simulink model "OtterFullForLqr_PositionControl_KALMAN"  (R2020b)
settings: Solver=ode4  StartTime=0.0  StopTime=100  FixedStep=0.01  RelTol=1e-3
model workspace (MAT data in the model file):
  count = 1
values from neighbouring files (symbols this model uses):
  u0 = [60 60]'    [LinMod60rpmForLqr.m]
  x0 = OpTrim60.states.x    [LinMod60rpmForLqr.m]
undefined symbols (not defined in the file or in its folder): F, N
libraries: mssSimulink x2, simulink x1
settings Model: Creator=rapha  LastModifiedBy=rapha
settings DataIOCC: ExternalInput=getinputstruct(op_trim1)  InitialState=getstatestruct(op_trim1)

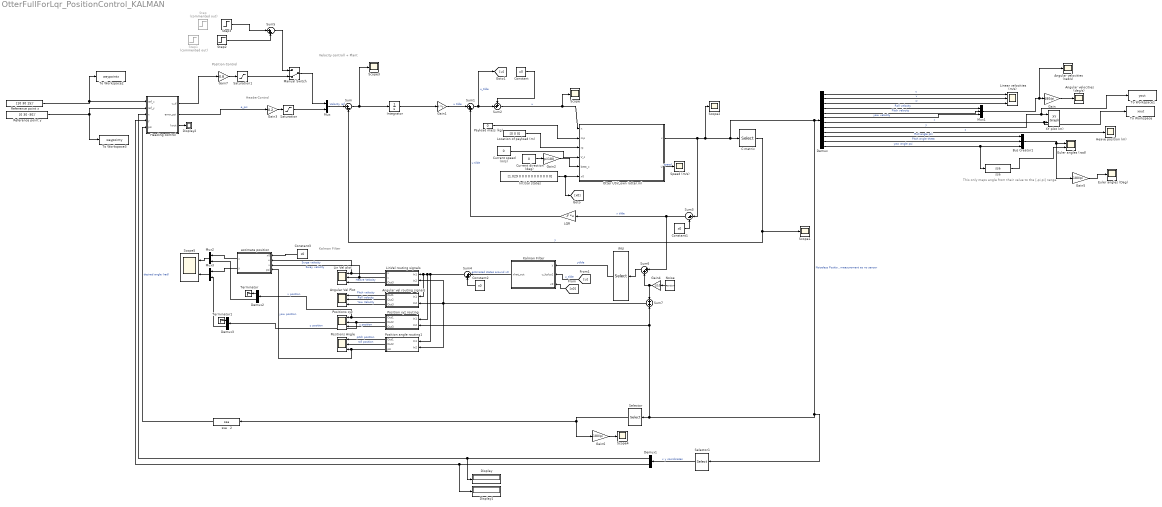
== system OtterFullForLqr_PositionControl_KALMAN ==
  note: Kalman Filter
  note: Position Control
  note: Velocity controll + Plant
  note: This only maps angle from their value to the [-pi,pi] range.
  note: HeaderControl
  Angular Vel Plot : Scope  NumInputPorts=3
  Angular vel routing signals : Subsystem
  Angular velocities (deg/s) : Scope
  Angular velocities (rad/s) : Scope
  Bus Creator1 : BusCreator  Inputs=3
  C matrix : Selector  InputPortWidth=12  IndexOptions=Index vector (dialog)  Indices=[1 6]  OutputSizes=1
  Constant : Constant  Value=u0
  Constant1 : Constant  Value=x0
  Constant2 : Constant  Value=x0
  Constant3 : Constant  Value=x0
  Current direction (deg) : Constant  Value=0
  Current speed (m/s) : Constant  Value=0
  Demux : Demux  Outputs=12
  Demux1 : Demux  Outputs=2
  Demux2 : Demux  Outputs=2
  Demux3 : Demux  Outputs=2
  Display : Display
  Display1 : Display
  Display2 : Display
  Euler angles (Deg) : Scope
  Euler angles (rad) : Scope  NumInputPorts=2
  Gain : Gain  Gain=180/pi
  Gain1 : Gain  Gain=N  Multiplication=Matrix(K*u)
  Gain2 : Gain  Gain=pi/180
  Gain3 : Gain  Gain=0.2
  Gain4 : Gain  Gain=1/10
  Gain5 : Gain  Gain=180/pi
  Gain6 : Gain  Gain=180/pi
  Gain7 : Gain  Gain=0.8
  Heading control : MATLAB Function  TreatAsAtomicUnit=on
  Heave position (m) : Scope
  IMU : Selector  InputPortWidth=12  IndexOptions=Index vector (dialog)  Indices=[1 2 3 4 5 6 10 11 12]  OutputSizes=1
  Integrator : Integrator
  Intitial states : Constant  Value=[1.029 0 0 0 0 0 0 0 0 0 0 0]
  Kalman Filter : MATLAB Function  TreatAsAtomicUnit=on
  LQR : Gain  Gain=-F  Multiplication=Matrix(K*u)
  Lin Vel plot : Scope  NumInputPorts=3
  LinVel routing signals : Subsystem
  Linear velocities (m/s) : Scope  NumInputPorts=3
  Location of payload (m) : Constant  Value=[0 0 0]
  Manual Switch : ManualSwitch  CurrentSetting=0
  Mux : Mux  Inputs=2
  Mux1 : Mux  Inputs=3
  Mux2 : Mux  Inputs=2
  Mux3 : Mux  Inputs=2
  Noise : RandomNumber  Variance=0.01  SampleTime=0.01
  "Otter USV_own (otter.m) " : Subsystem  AncestorBlock=mssSimulink/Marine craft models/Otter USV (otter.m)
      mask Display: image('otter.jpg'); % Use "Edit Image" on toolstrip to change.
  Payload mass (kg) : Constant  Value=0
  Position angle routing1 : Subsystem
  Position xyz routing : Subsystem
  Positions Angle : Scope  NumInputPorts=3
  Positions xyz : Scope  NumInputPorts=3
  Reference point x : Constant  Value=[10 30 15]'
  Reference point y : Constant  Value=[0 30 -30]'
  Saturation : Saturate
  Saturation1 : Saturate  UpperLimit=1.5  LowerLimit=-1.5
  Scope{,1..4} (5 alike) : Scope
  Scope5 : Scope  NumInputPorts=2
  Selector : Selector  InputPortWidth=12  IndexOptions=Index vector (dialog)  Indices=[12]  OutputSizes=1
  Selector1 : Selector  InputPortWidth=12  IndexOptions=Index vector (dialog)  Indices=[7 8]  OutputSizes=1
  Speed (m/s) : Scope
  Step : Step  Commented=on  Before=0.5  After=0.5  SampleTime=0
  Step1 : Step  Commented=on  After=90  SampleTime=0
  Step2 : Step  Time=10  Before=1.029  After=0.8  SampleTime=0
  Step3 : Step  Time=15  After=0.3  SampleTime=0
  Sum : Sum  Inputs=|+-
  Sum{1,4..6} (4 alike) : Sum  Inputs=|++
  Sum2 : Sum  Inputs=++|
  Sum3 : Sum  Inputs=|+-
  Sum7 : Sum  Inputs=+|+
  Terminator : Terminator
  Terminator1 : Terminator
  To Workspace : ToWorkspace  VariableName=xout  SampleTime=-1
  To Workspace1 : ToWorkspace  VariableName=yout  SampleTime=-1
  To Workspace2 : ToWorkspace  VariableName=waypointx  SampleTime=-1
  To Workspace3 : ToWorkspace  VariableName=waypointy  SampleTime=-1
  XY plot (m) : simulink/Sinks/XY Graph  xmin=-70  xmax=70  ymin=-70  ymax=70  st=0.01
  estimate position : MATLAB Function  TreatAsAtomicUnit=on
  "ssa   " : mssSimulink/Utilities/Math Operations/ssa  SystemSampleTime=-1  VariantActivationTime=update diagram  Latency=0  AutoFrameSizeCalculation=off
  ssa   2 : mssSimulink/Utilities/Math Operations/ssa  SystemSampleTime=-1  VariantActivationTime=update diagram  Latency=0  AutoFrameSizeCalculation=off
  wires:
  Intitial states/1 -> [x0], "Otter USV_own (otter.m) "/6(x0)
  Payload mass (kg)/1 -> "Otter USV_own (otter.m) "/2(mp)
  Gain2/1 -> "Otter USV_own (otter.m) "/5(beta_c)
  Current direction (deg)/1 -> Gain2/1
  "Otter USV_own (otter.m) "/2(U) -> Speed (m/s)/1  "speed"
  Current speed (m/s)/1 -> "Otter USV_own (otter.m) "/4(V_c)
  Location of payload (m)/1 -> "Otter USV_own (otter.m) "/3(rp)
  Demux/1 -> Linear velocities (m/s)/1  "u"
  Demux/8 -> XY plot (m)/1, To Workspace1/1  "y"
  Demux/7 -> To Workspace/1, XY plot (m)/2  "x"
  Demux/2 -> Linear velocities (m/s)/2  "v"
  Demux/3 -> Linear velocities (m/s)/3  "w"
  Gain/1 -> Angular velocities (deg/s)/1
  Mux1/1 -> Angular velocities (rad/s)/1, Gain/1
  Demux/4 -> Mux1/1  "Roll velocity"
  Demux/5 -> Mux1/2  "Pitch velocity"
  Demux/6 -> Mux1/3  "yaw velocity"
  Demux/9 -> Heave position (m)/1  "z"
  Demux/11 -> Bus Creator1/2  "Pitch angle theta"
  Bus Creator1/1 -> Euler angles (rad)/1, Gain5/1
  Demux/10 -> Bus Creator1/1  "Roll angle phi"
  Demux/12 -> "ssa   "/1, Bus Creator1/3  "yaw angle psi"
  "ssa   "/1 -> Euler angles (rad)/2
  "Otter USV_own (otter.m) "/1(x) -> Sum3/1, Demux/1, Selector1/1, Selector/1, Position xyz routing/2(In2), Sum7/2, C matrix/1, Scope2/1  "Noiseless Position measurement as no sensor"
  C matrix/1 -> Sum/2, Scope1/1  "y"
  Sum/1 -> Integrator/1, Scope3/1
  LQR/1 -> Sum1/2  "u tilde"
  Gain1/1 -> Sum1/1  "u tilde"
  Sum2/1 -> Scope/1, "Otter USV_own (otter.m) "/1(n)  "u"
  Sum3/1 -> LQR/1, Sum6/1  "x tilde"
  Constant1/1 -> Sum3/2
  Constant/1 -> Sum2/1
  Integrator/1 -> Gain1/1
  Mux/1 -> Sum/1  "Velocity ref"
  Gain5/1 -> Euler angles (Deg)/1
  Gain6/1 -> Scope4/1
  Reference point x/1 -> To Workspace2/1, Heading control/1(ref_x)
  Selector1/1 -> Demux1/1  "x y coordinates"
  Demux1/1 -> Display/1, Heading control/3(x)
  Demux1/2 -> Display1/1, Heading control/4(y)
  Gain7/1 -> Saturation1/1
  Heading control/1(u_d) -> Gain7/1
  Reference point y/1 -> Heading control/2(ref_y), To Workspace3/1
  Heading control/3(kout) -> Display2/1
  Selector/1 -> Gain6/1, ssa   2/1
  Saturation/1 -> Mux/2
  Gain3/1 -> Saturation/1
  Heading control/2(error_psi) -> Gain3/1  "e_psi"
  ssa   2/1 -> Heading control/5(psi)  "desired angle (rad)"
  [x0] -> Kalman Filter/3(x0)
  [u] -> Kalman Filter/2(u_kplus1)  "u_tilde"
  IMU/1 -> Kalman Filter/1(y)  "ytilde"
  Sum1/1 -> [u], Sum2/2  "u_tilde"
  Saturation1/1 -> Manual Switch/2
  Manual Switch/1 -> Mux/1
  Kalman Filter/1(xhat_out) -> Sum4/1  "estimated states around x0"
  Sum4/1 -> Position angle routing1/1(In1), Position xyz routing/1(In1), Angular vel routing signals/1(In1), LinVel routing signals/1(In1)
  Constant2/1 -> Sum4/2
  Step2/1 -> Sum5/2
  Sum5/1 -> Manual Switch/1
  Step3/1 -> Sum5/1
  LinVel routing signals/1(u) -> estimate position/2(u), Lin Vel plot/1  "Surge velocity"
  LinVel routing signals/2(v) -> Lin Vel plot/2, estimate position/3(v)  "Sway velocity"
  LinVel routing signals/3(Out3) -> Lin Vel plot/3  "Heave Velocity"
  Sum6/1 -> IMU/1
  Noise/1 -> Gain4/1
  Gain4/1 -> Sum6/2, Sum7/1
  Sum7/1 -> LinVel routing signals/2(In2), Position angle routing1/2(In2), Angular vel routing signals/2(In2)
  Angular vel routing signals/2(Out2) -> Angular Vel Plot/2  "Roll velocity"
  Angular vel routing signals/3(Out3) -> Angular Vel Plot/3  "Yaw Velocity"
  Angular vel routing signals/1(Out1) -> Angular Vel Plot/1  "Pitch velocity"
  Position xyz routing/1(Out1) -> Demux2/1, Positions xyz/1  "x position"
  Position xyz routing/3(Out3) -> Positions xyz/3  "z position"
  Position angle routing1/3(psi) -> estimate position/4(psi), Positions Angle/3  "yaw position"
  Position angle routing1/2(Out2) -> Positions Angle/2  "roll position"
  Position angle routing1/1(Out1) -> Positions Angle/1  "pitch position"
  Constant3/1 -> estimate position/1(x0)
  Mux2/1 -> Scope5/1
  estimate position/1(x) -> Mux2/1
  Mux3/1 -> Scope5/2
  estimate position/2(y) -> Mux3/1
  Demux2/2 -> Mux2/2
  Demux3/2 -> Mux3/2
  Position xyz routing/2(Out2) -> Demux3/1, Positions xyz/2  "y position"
  Demux2/1 -> Terminator/1
  Demux3/1 -> Terminator1/1

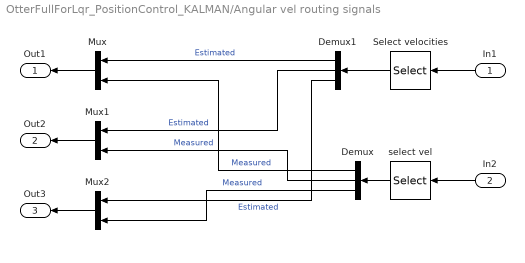
== system OtterFullForLqr_PositionControl_KALMAN/Angular vel routing signals ==
  In1 : Inport
  In2 : Inport  Port=2
  Demux : Demux  Outputs=3
  Demux1 : Demux  Outputs=3
  Mux : Mux  Inputs=2
  Mux1 : Mux  Inputs=2
  Mux2 : Mux  Inputs=2
  Select velocities : Selector  InputPortWidth=12  IndexOptions=Index vector (dialog)  Indices=[4 5 6]  OutputSizes=1
  select vel : Selector  InputPortWidth=12  IndexOptions=Index vector (dialog)  Indices=[4 5 6]  OutputSizes=1
  Out1 : Outport
  Out2 : Outport  Port=2
  Out3 : Outport  Port=3
  wires:
  In2/1 -> select vel/1
  In1/1 -> Select velocities/1
  select vel/1 -> Demux/1
  Select velocities/1 -> Demux1/1
  Mux/1 -> Out1/1
  Mux1/1 -> Out2/1
  Mux2/1 -> Out3/1
  Demux1/1 -> Mux/1  "Estimated"
  Demux/1 -> Mux/2  "Measured"
  Demux1/2 -> Mux1/1  "Estimated"
  Demux/2 -> Mux1/2  "Measured"
  Demux1/3 -> Mux2/1  "Estimated"
  Demux/3 -> Mux2/2  "Measured"

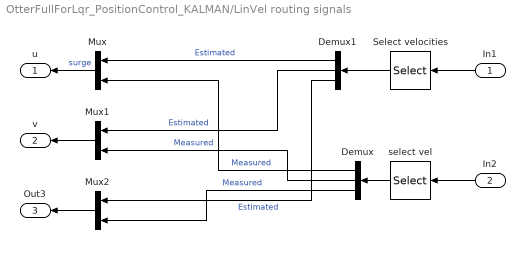
== system OtterFullForLqr_PositionControl_KALMAN/LinVel routing signals ==
  In1 : Inport
  In2 : Inport  Port=2
  Demux : Demux  Outputs=3
  Demux1 : Demux  Outputs=3
  Mux : Mux  Inputs=2
  Mux1 : Mux  Inputs=2
  Mux2 : Mux  Inputs=2
  Select velocities : Selector  InputPortWidth=12  IndexOptions=Index vector (dialog)  Indices=[1 2 3]  OutputSizes=1
  select vel : Selector  InputPortWidth=12  IndexOptions=Index vector (dialog)  Indices=[1 2 3]  OutputSizes=1
  u : Outport
  v : Outport  Port=2
  Out3 : Outport  Port=3
  wires:
  In2/1 -> select vel/1
  In1/1 -> Select velocities/1
  select vel/1 -> Demux/1
  Select velocities/1 -> Demux1/1
  Mux/1 -> u/1  "surge"
  Mux1/1 -> v/1
  Mux2/1 -> Out3/1
  Demux1/1 -> Mux/1  "Estimated"
  Demux/1 -> Mux/2  "Measured"
  Demux1/2 -> Mux1/1  "Estimated"
  Demux/2 -> Mux1/2  "Measured"
  Demux1/3 -> Mux2/1  "Estimated"
  Demux/3 -> Mux2/2  "Measured"

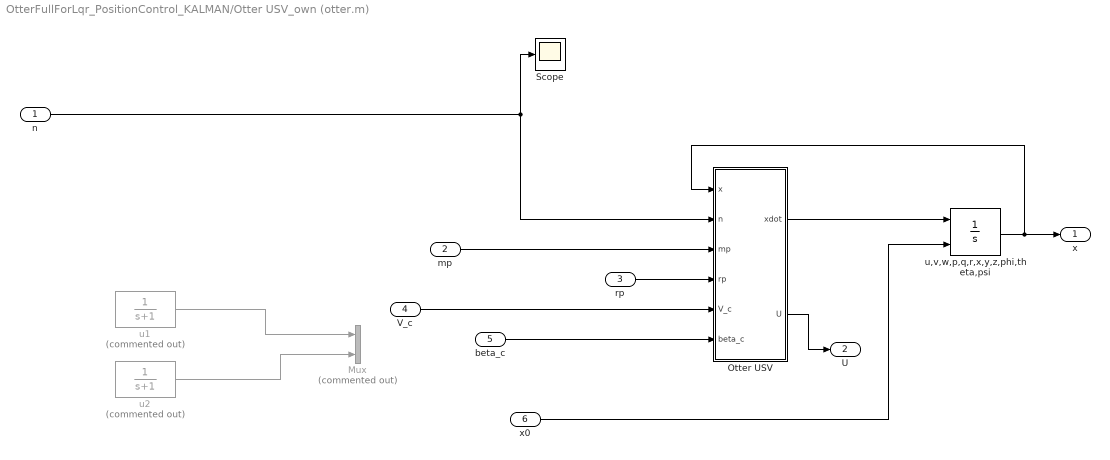
== system OtterFullForLqr_PositionControl_KALMAN/Otter USV_own (otter.m)  ==
  n : Inport
  mp : Inport  Port=2
  rp : Inport  Port=3
  V_c : Inport  Port=4
  beta_c : Inport  Port=5
  x0 : Inport  Port=6
  Mux : Mux  Commented=on  Inputs=2
  Otter USV : MATLAB Function  TreatAsAtomicUnit=on
  Scope : Scope
  u,v,w,p,q,r,x,y,z,phi,theta,psi : Integrator  InitialConditionSource=external  InitialCondition=[1 1]  UpperSaturationLimit=10  LowerSaturationLimit=-10  AbsoluteTolerance=1e-3
  u1 : TransferFcn  Commented=on  Denominator=[1 1]
  u2 : TransferFcn  Commented=on  Denominator=[1 1]
  x : Outport
  U : Outport  Port=2
  wires:
  V_c/1 -> Otter USV/5(V_c)
  Otter USV/2(U) -> U/1
  mp/1 -> Otter USV/3(mp)
  Otter USV/1(xdot) -> u,v,w,p,q,r,x,y,z,phi,theta,psi/1
  u,v,w,p,q,r,x,y,z,phi,theta,psi/1 -> Otter USV/1(x), x/1
  beta_c/1 -> Otter USV/6(beta_c)
  rp/1 -> Otter USV/4(rp)
  x0/1 -> u,v,w,p,q,r,x,y,z,phi,theta,psi/2
  n/1 -> Scope/1, Otter USV/2(n)
  u2/1 -> Mux/2
  u1/1 -> Mux/1

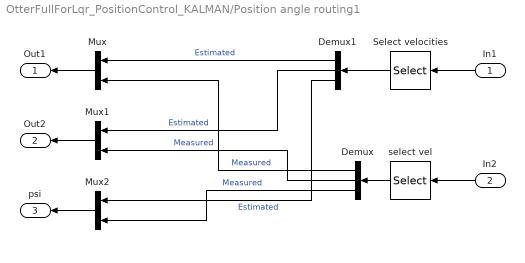
== system OtterFullForLqr_PositionControl_KALMAN/Position angle routing1 ==
  In1 : Inport
  In2 : Inport  Port=2
  Demux : Demux  Outputs=3
  Demux1 : Demux  Outputs=3
  Mux : Mux  Inputs=2
  Mux1 : Mux  Inputs=2
  Mux2 : Mux  Inputs=2
  Select velocities : Selector  InputPortWidth=12  IndexOptions=Index vector (dialog)  Indices=[10 11 12]  OutputSizes=1
  select vel : Selector  InputPortWidth=12  IndexOptions=Index vector (dialog)  Indices=[10 11 12]  OutputSizes=1
  Out1 : Outport
  Out2 : Outport  Port=2
  psi : Outport  Port=3
  wires:
  In2/1 -> select vel/1
  In1/1 -> Select velocities/1
  select vel/1 -> Demux/1
  Select velocities/1 -> Demux1/1
  Mux/1 -> Out1/1
  Mux1/1 -> Out2/1
  Mux2/1 -> psi/1
  Demux1/1 -> Mux/1  "Estimated"
  Demux/1 -> Mux/2  "Measured"
  Demux1/2 -> Mux1/1  "Estimated"
  Demux/2 -> Mux1/2  "Measured"
  Demux1/3 -> Mux2/1  "Estimated"
  Demux/3 -> Mux2/2  "Measured"

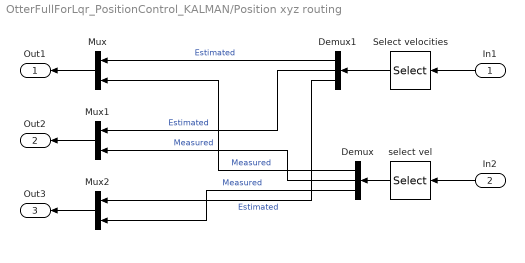
== system OtterFullForLqr_PositionControl_KALMAN/Position xyz routing ==
  In1 : Inport
  In2 : Inport  Port=2
  Demux : Demux  Outputs=3
  Demux1 : Demux  Outputs=3
  Mux : Mux  Inputs=2
  Mux1 : Mux  Inputs=2
  Mux2 : Mux  Inputs=2
  Select velocities : Selector  InputPortWidth=12  IndexOptions=Index vector (dialog)  Indices=[7 8 9]  OutputSizes=1
  select vel : Selector  InputPortWidth=12  IndexOptions=Index vector (dialog)  Indices=[7 8 9]  OutputSizes=1
  Out1 : Outport
  Out2 : Outport  Port=2
  Out3 : Outport  Port=3
  wires:
  In2/1 -> select vel/1
  In1/1 -> Select velocities/1
  select vel/1 -> Demux/1
  Select velocities/1 -> Demux1/1
  Mux/1 -> Out1/1
  Mux1/1 -> Out2/1
  Mux2/1 -> Out3/1
  Demux1/1 -> Mux/1  "Estimated"
  Demux/1 -> Mux/2  "Measured"
  Demux1/2 -> Mux1/1  "Estimated"
  Demux/2 -> Mux1/2  "Measured"
  Demux1/3 -> Mux2/1  "Estimated"
  Demux/3 -> Mux2/2  "Measured"

== matlab function OtterFullForLqr_PositionControl_KALMAN/Heading control ==
  settings: updateMethod=DISCRETE
  data: ref_x input; ref_y input; u_d output; x input; error_psi output; y input; psi input; kout output
function [u_d,error_psi,kout] = fcn(ref_x,ref_y,x,y,psi)
%% Initialize the ref point we want to track
Npoint=size(ref_x,1);
persistent k;

if isempty(k)
    k=1;
end
kout=k;
if (k<=Npoint)

    x_ref=ref_x(k);
    y_ref=ref_y(k);
    
    %% Compute desired yaw angle
    psi_d = atan2(y_ref-y, x_ref-x);  % Calculate the angle between the two points
    %% Error calculation
    error_psi=psi_d-psi;
    error_dist=sqrt((y_ref-y)^2+(x_ref-x)^2);
    %% Control law for psi = INNER LOOP
    % Mapping to avoid dicontinuities when crossing pi or -pi.
    if(error_psi<-pi)
        error_psi=error_psi+2*pi;
    elseif (error_psi>=pi)
        error_psi=error_psi-2*pi;
    end
    %% Compute surge velocity wished depending on the boat orientation.=OUTERLOOP
    if (abs(error_dist)>1 && abs(error_psi)<7*(pi/180)) %When far away from set point and angle is already close to the wished one
        u_d=error_dist;
    elseif(abs(error_dist)<1)
        k=k+1;
        u_d=error_dist/10;
    else
        u_d=error_dist/100;%Move slowly when close to the point or if the angle error is too big.
    end
else
    u_d=0;
    error_psi=0;
end

== matlab function OtterFullForLqr_PositionControl_KALMAN/Otter USV_own (otter.m) /Otter USV ==
  settings: updateMethod=DISCRETE
  data: x input; n input; xdot output; mp input; rp input; V_c input; beta_c input; U output
function [xdot,U] = fcn(x,n,mp,rp,V_c,beta_c)

[xdot,U] = OtterFunction_lqr(x,n,mp,rp,V_c,beta_c);

end

== matlab function OtterFullForLqr_PositionControl_KALMAN/Kalman Filter ==
  settings: updateMethod=DISCRETE
  data: y input; u_kplus1 input; xhat_out output; x0 input
function xhat_out = fcn(y,u_kplus1,x0)
%% Linear model 
persistent P
persistent u_k
persistent xhat_k

A=[-1.3626   -0.0000   -0.0187   -0.0000   -1.3495   -0.0000         0         0  -12.1557         0  -16.1415         0;
    0.0000   -0.0000   -0.0000    0.2504    0.0000   -0.3477         0         0         0    4.9601         0         0;
   -0.0417   -0.0000   -4.9783    0.0000   -0.1756   -0.0000         0         0  -75.2200         0  -22.5575         0;
   -0.0000    0.0000   -0.0000   -3.3993    0.0000   -0.1414         0         0         0  -67.3414         0         0;
   -0.4167   -0.0000   -0.1027   -0.0000   -7.3953   -0.0000         0         0  -66.6151         0  -88.4576         0;
    0.0000    0.0000   -0.0000    0.2696    0.0000   -1.1519         0         0         0    5.3406         0         0;
    1.0000         0   -0.0000         0         0         0         0         0         0         0    0.0000         0;
         0    1.0000   -0.0000         0         0         0         0         0         0    0.0000         0    1.0290;
    0.0000    0.0000    1.0000         0         0         0         0         0         0         0   -1.0290         0;
         0         0         0    1.0000         0   -0.0000         0         0         0   -0.0000    0.0000         0;
         0         0         0         0    1.0000   -0.0000         0         0         0         0         0         0;
         0         0         0         0    0.0000    1.0000         0         0         0    0.0000   -0.0000         -4];

B= [0.0234    0.0234;
   -0.0008    0.0008;
    0.0007    0.0007;
   -0.0026    0.0026;
    0.0071    0.0071;
    0.0120   -0.0120;
         0         0;
         0         0;
         0         0;
         0         0;
         0         0;
         0         0];
     
C=[1 0 0 0 0 0 0 0 0 0 0 0
   0 1 0 0 0 0 0 0 0 0 0 0
   0 0 1 0 0 0 0 0 0 0 0 0 
   0 0 0 1 0 0 0 0 0 0 0 0
   0 0 0 0 1 0 0 0 0 0 0 0
   0 0 0 0 0 1 0 0 0 0 0 0
   0 0 0 0 0 0 0 0 0 1 0 0
   0 0 0 0 0 0 0 0 0 0 1 0
   0 0 0 0 0 0 0 0 0 0 0 1];

%% Equilibrium point
u_eq=[60 60]';
x_eq=[1.029;
         0;
       0.0;
       0.0;
       0.0;
       0.0;
       0.0;
       0.0;
       0.0;
       0.0;
       0.0;
       0.0];

% y_k+1 is y in this code, as coming from simulink

%% Initialization
if isempty(P)
    P=zeros(12,12); %only valid if we know initial position before predicting.
end
if isempty(u_k)
    u_k=u_eq;
end

if isempty(xhat_k)
    xhat_k=x0;  %initial guess of the position. Assumed to be known so P matrix start at zero(12,12)
end
% sigma=1e-1;
Q = eye(12)*100; %should be same size as P and A
R = eye(9)*1; % CPC gives a 2x2 matrix

%% Kalman Filter
%prediction
xhat_kplus1= A*xhat_k+B*u_k;
P = A*P*A' + Q;
%correction
K = P*C'*(C*P*C'+R)^(-1);
xhat_kplus1=xhat_kplus1+K*(y-C*xhat_kplus1);%recompute hat_x(k) to correct with output values.
P=P-K*C*P;

%% Set u value for next iteration, where we need uk and not uk+1
u_k=u_kplus1; 
xhat_k=xhat_kplus1; % For next iteration xk.
xhat_out=xhat_kplus1;

== matlab function OtterFullForLqr_PositionControl_KALMAN/estimate position ==
  settings: updateMethod=DISCRETE
  data: x output; x0 input; u input; v input; y output; psi input
function [x,y] = EstimatePosition(x0,u,v,psi)
persistent x_prev
persistent y_prev
if isempty(x_prev)
    x_prev=x0(7);
end
if isempty(y_prev)
    y_prev=x0(8);
end
h=0.01;
V=sqrt(u(1)^2+v(1)^2); %get forward verctor speed, pytagore
x=(cos(psi(1))*V)*h+x_prev;
y=(sin(psi(1))*V)*h+y_prev;

x_prev=x;
y_prev=y;
